simulink model "ps5"  (R2020b)
settings: Solver=VariableStepAuto  StartTime=0.0  StopTime=10.0  RelTol=1e-3
model workspace (MAT data in the model file):
  C = 1e-05
  R = 10
settings Model: Creator=prana  LastModifiedBy=prana

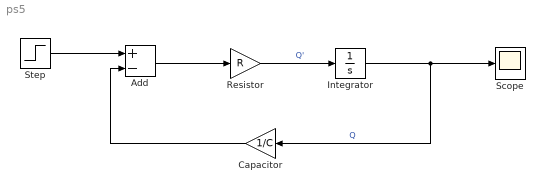
== system ps5 ==
  Add : Sum  Inputs=+-
  Capacitor : Gain  Gain=1/C
  Integrator : Integrator
  Resistor : Gain  Gain=R
  Scope : Scope
  Step : Step  SampleTime=0
  wires:
  Step/1 -> Add/1
  Add/1 -> Resistor/1
  Resistor/1 -> Integrator/1  "Q'"
  Integrator/1 -> Scope/1, Capacitor/1  "Q"
  Capacitor/1 -> Add/2
